simulink subsystem "dynamics_sub"  (R2022b)
settings: Solver=VariableStepAuto  StartTime=0.0  StopTime=10.0  RelTol=1e-3
libraries: dspsigops x1
settings Model: Creator=gotta  LastModifiedBy=giuliapegoraro

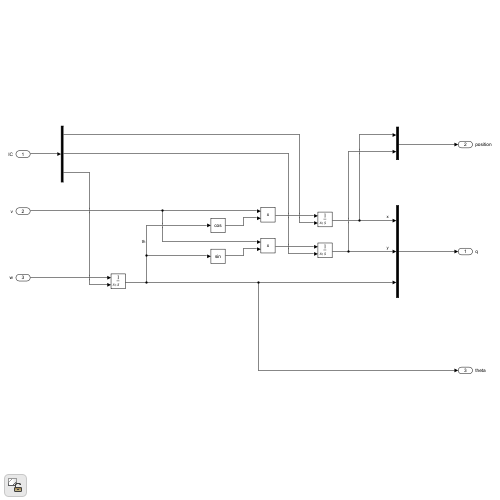
[thumbnail: Simulink's stored preview of the top-level diagram]
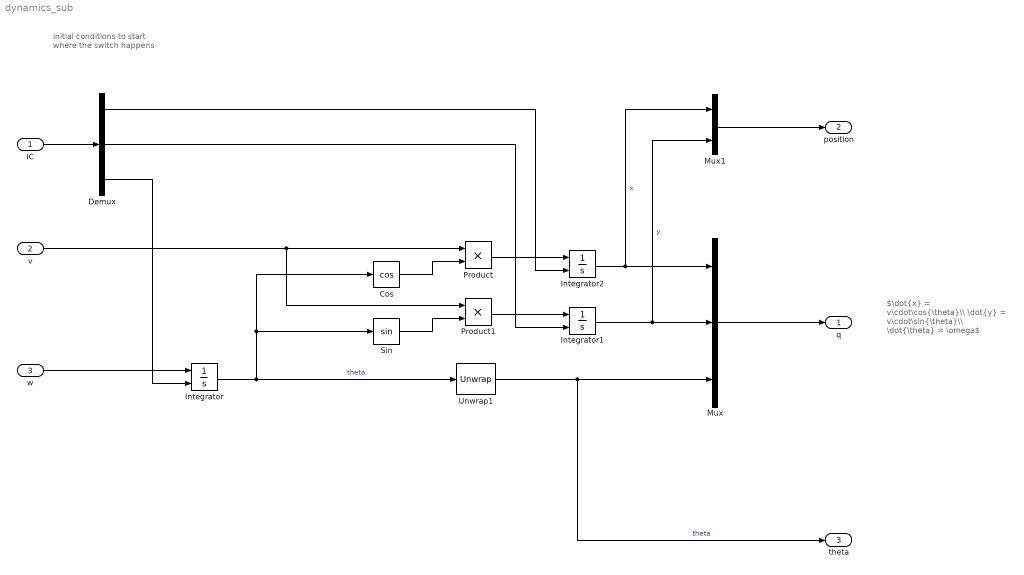
== system dynamics_sub ==
  note: $\dot{x} = v\cdot\cos{\theta}\\ \dot{y} = v\cdot\sin{\theta}\\ \dot{\theta} = \omega$
  note: initial conditions to start
      | where the switch happens
  IC : Inport
  v : Inport  Port=2
  w : Inport  Port=3
  Cos : Trigonometry  Operator=cos
  Demux : Demux  Outputs=3
  Integrator : Integrator  InitialConditionSource=external
  Integrator1 : Integrator  InitialConditionSource=external
  Integrator2 : Integrator  InitialConditionSource=external
  Mux : Mux  Inputs=3
  Mux1 : Mux  Inputs=2
  Product : Product
  Product1 : Product
  Sin : Trigonometry
  Unwrap1 : dspsigops/Unwrap  tol=pi  InputProcessing=Columns as channels (frame based)  running=off
  q : Outport
  position : Outport  Port=2
  theta : Outport  Port=3
  wires:
  Demux/3 -> Integrator/2
  Demux/2 -> Integrator1/2
  Demux/1 -> Integrator2/2
  IC/1 -> Demux/1
  Cos/1 -> Product/2
  Integrator2/1 -> Mux/1, Mux1/1  "x"
  Sin/1 -> Product1/2
  Integrator1/1 -> Mux1/2, Mux/2  "y"
  Integrator/1 -> Unwrap1/1, Sin/1, Cos/1  "theta"
  Product1/1 -> Integrator1/1
  Product/1 -> Integrator2/1
  v/1 -> Product1/1, Product/1
  w/1 -> Integrator/1
  Mux/1 -> q/1
  Mux1/1 -> position/1
  Unwrap1/1 -> theta/1, Mux/3  "theta"
